simulink model "Model_OnlyDark_17_09_07_hperrorsign_manyouts"  (R2015a)
settings: Solver=FixedStepDiscrete  StartTime=0.0  StopTime=60  FixedStep=0.05  RelTol=1e-3
InitFcn:
  | %Ts=parameter.Ts;
  |    %Sampling Time, 50 times slower than original model
model workspace (MAT data in the model file):
  padsize = 8
  x1 = 14
undefined symbols (not defined in the file): alpha_downslope_off, alpha_downslope_on, alpha_upslope_off, alpha_upslope_on, fdsr_lp, hdegs, TimeStep, vdegs
libraries: visionfilter x3, visionutilities x3
settings Model: tstep=0.1  TimeStep=0.1  CovSFcnEnable=off  Creator=a1174239  LastModifiedBy=John
settings SolverCC: AlgebraicLoopSolver=LineSearch
settings DataIOCC: MaxDataPoints=1
settings OptimizationCC: ExpressionDepthLimit=2147483647  EfficientMapNaN2IntZero=off
settings DebuggingCC: UnderspecifiedInitializationDetection=Classic  MergeDetectMultiDrivingBlocksExec=none  SolverPrmCheckMsg=warning  MultiTaskDSMMsg=warning  MultiTaskCondExecSysMsg=none  ParameterPrecisionLossMsg=none  StateNameClashWarn=warning
settings HardwareCC: TargetLongLongMode=on  TargetIntDivRoundTo=Zero  TargetEndianess=LittleEndian  TargetHWDeviceType=MATLAB Host  ProdEqTarget=off
settings CodeAppCC: MaxIdLength=128
settings GRTTargetCC: CombineOutputUpdateFcns=off  GRTInterface=on

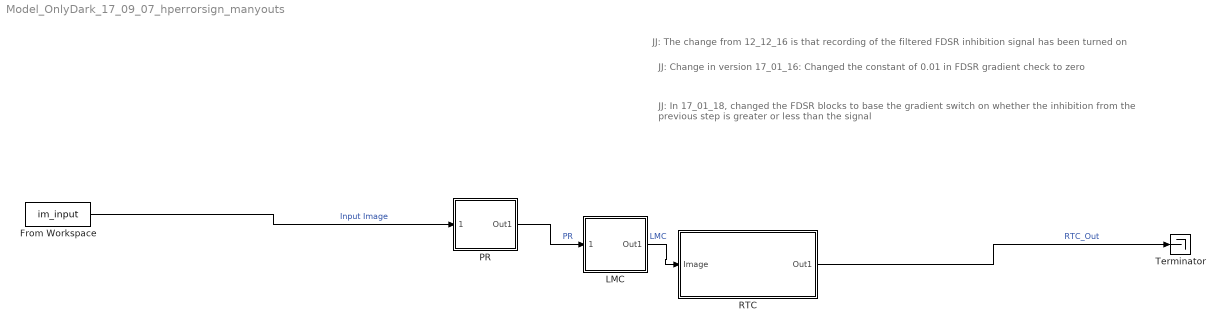
== system Model_OnlyDark_17_09_07_hperrorsign_manyouts ==
  note: JJ: In 17_01_18, changed the FDSR blocks to base the gradient switch on whether the inhibition from the previous step is greater or less than the signal
  note: JJ: Change in version 17_01_16: Changed the constant of 0.01 in FDSR gradient check to zero
  note: JJ: The change from 12_12_16 is that recording of the filtered FDSR inhibition signal has been turned on
  From Workspace : FromWorkspace  VariableName=im_input  SampleTime=0.001  Interpolate=off  OutputAfterFinalValue=Holding final value
  LMC : Subsystem
  PR : Subsystem
  RTC : Subsystem
  Terminator : Terminator
  wires:
  PR/1(Out1) -> LMC/1(Image)  "PR"
  LMC/1(Out1) -> RTC/1(Image)  "LMC"
  RTC/1(Out1) -> Terminator/1  "RTC_Out"
  From Workspace/1 -> PR/1(Image)  "Input Image"

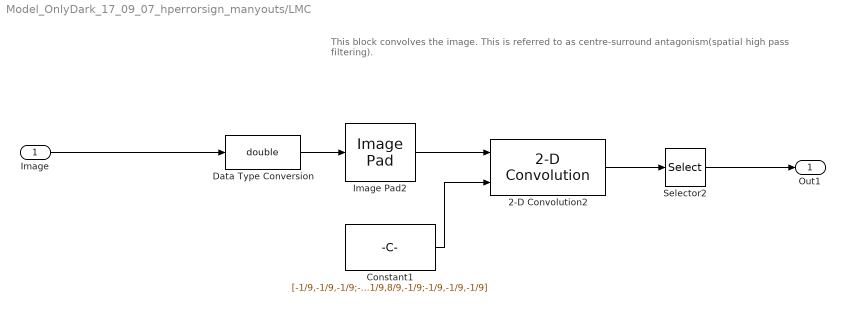
== system Model_OnlyDark_17_09_07_hperrorsign_manyouts/LMC ==
  note: This block convolves the image. This is referred to as centre-surround antagonism(spatial high pass filtering).
  Image : Inport
  2-D Convolution2 : visionfilter/2-D Convolution  outSize=Same as input port I1  normalize=off  outputMode=Binary point scaling  outputWordLength=32  outputFracLength=12  prodOutputMode=Binary point scaling  prodOutputWordLength=32  prodOutputFracLength=10  roundingMode=Floor  overflowMode=off
  Constant1 : Constant  Value=[-1/9,-1/9,-1/9;-1/9,8/9,-1/9;-1/9,-1/9,-1/9]
  Data Type Conversion : DataTypeConversion  OutDataTypeStr=double
  Image Pad2 : visionutilities/Image Pad  method=Symmetric  valSrc=Specify via dialog  value=0  spec=Pad size  rowDirection=Both left and right  outRowsMode=User-specified  rowSize=1  outColSize=10  colDirection=Both top and bottom  outColsMode=User-specified  colSize=1  outRowSize=12  trunc_flag=None
  Selector2 : Selector  NumberOfDimensions=2  InputPortWidth=3  IndexOptions=Index vector (dialog),Index vector (dialog)  Indices=[2:vdegs+1],[2:hdegs+1]  OutputSizes=1,1
  Out1 : Outport
  wires:
  Constant1/1 -> 2-D Convolution2/2
  Image Pad2/1 -> 2-D Convolution2/1
  2-D Convolution2/1 -> Selector2/1
  Selector2/1 -> Out1/1
  Image/1 -> Data Type Conversion/1
  Data Type Conversion/1 -> Image Pad2/1

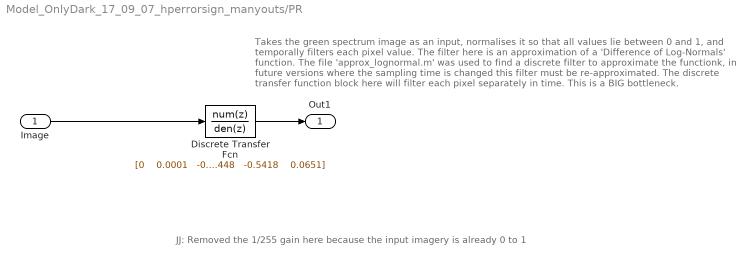
== system Model_OnlyDark_17_09_07_hperrorsign_manyouts/PR ==
  note: JJ: Removed the 1/255 gain here because the input imagery is already 0 to 1
  note: Takes the green spectrum image as an input, normalises it so that all values lie between 0
      | and 1, and temporally filters each pixel value. The filter here is an approximation of a
      | 'Difference of Log-Normals' function. The file 'approx_lognormal.m' was used to find a discrete
      | filter to approximate the functionk, in future versions where the sampling time is changed this filter
      | must be re-approximated.
      |
      | The discrete transfer function block here will filter each pixel separately in time. This is a BIG bottleneck.
  Image : Inport
  Discrete Transfer Fcn : DiscreteTransferFcn  Numerator="[0    0.0001   -0.0011    0.0052   -0.0170    0.0439   -0.0574    0.1789   -0.1524]"  Denominator="[ 1.0000   -4.3331    8.6847  -10.7116    9.0004   -5.3058    2.1448   -0.5418    0.0651]"
  Out1 : Outport
  wires:
  Image/1 -> Discrete Transfer Fcn/1
  Discrete Transfer Fcn/1 -> Out1/1

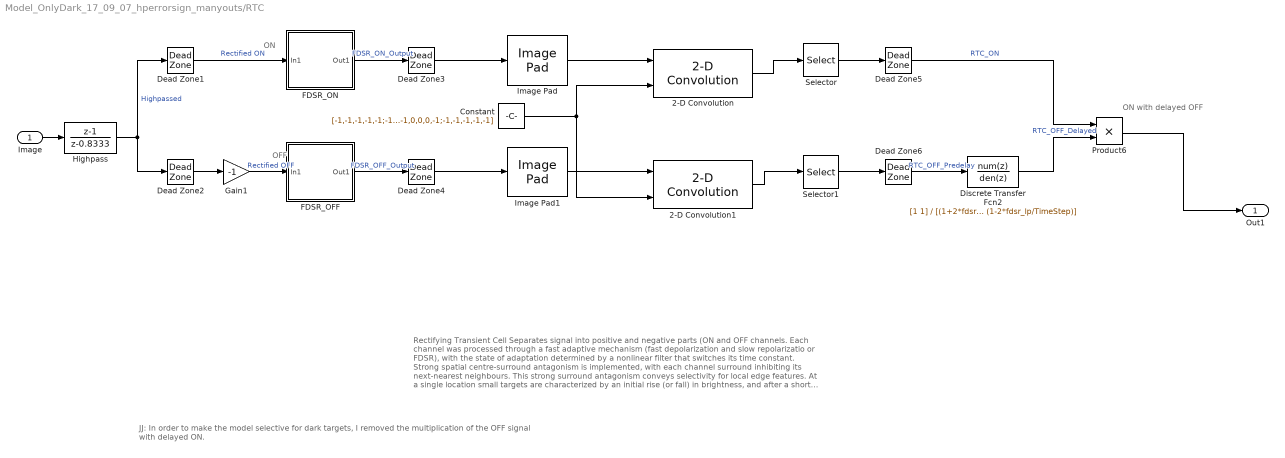
== system Model_OnlyDark_17_09_07_hperrorsign_manyouts/RTC ==
  note: ON with delayed OFF
  note: JJ: In order to make the model selective for dark targets, I removed the multiplication of the OFF signal with delayed ON.
  note: ON
  note: OFF
  note: Rectifying Transient Cell Separates signal into positive and negative parts (ON and OFF channels. Each channel was processed through a fast adaptive mechanism (fast depolarization and slow repolarizatio or FDSR),
      | with the state of adaptation determined by a nonlinear filter that switches its time constant. Strong spatial centre-surround antagonism is implemented, with each channel surround inhibiting its next-nearest neighbours.
      | This strong surround antagonism conveys selectivity for local edge features. At a single location small targets are characterized by an initial rise (or fall) in brightness, and after a short delay are followed by a corresponding
      | fall (or rise), irrespective of the direction of travel. Sensitivity to targets independent of their polarity was provided by multiplying each contrast channel (ON or OFF) with a delayed version of the opposite polarity
      | (via a low-pass filter,) and then summing the outputs.
  Image : Inport
  2-D Convolution : visionfilter/2-D Convolution  outSize=Same as input port I1  normalize=off  outputMode=Binary point scaling  outputWordLength=32  outputFracLength=12  prodOutputMode=Binary point scaling  prodOutputWordLength=32  prodOutputFracLength=10  roundingMode=Floor  overflowMode=off
  2-D Convolution1 : visionfilter/2-D Convolution  outSize=Same as input port I1  normalize=off  outputMode=Binary point scaling  outputWordLength=32  outputFracLength=12  prodOutputMode=Binary point scaling  prodOutputWordLength=32  prodOutputFracLength=10  roundingMode=Floor  overflowMode=off
  Constant : Constant  Value=[-1,-1,-1,-1,-1;-1,0,0,0,-1;-1,0,2,0,-1; -1,0,0,0,-1;-1,-1,-1,-1,-1]
  Dead Zone{1,3..6} (5 alike) : DeadZone  LowerValue=-inf  UpperValue=0  SaturateOnIntegerOverflow=on
  Dead Zone2 : DeadZone  LowerValue=0  UpperValue=inf  SaturateOnIntegerOverflow=on
  Discrete Transfer Fcn2 : DiscreteTransferFcn  Numerator=[1 1]  Denominator=[(1+2*fdsr_lp/TimeStep), (1-2*fdsr_lp/TimeStep)]
  FDSR_OFF : Subsystem
  FDSR_ON : Subsystem
  Gain1 : Gain  Gain=-1
  Highpass : DiscreteTransferFcn  Numerator=[1 -1]  Denominator=[1 -0.8333]
  Image Pad : visionutilities/Image Pad  method=Symmetric  valSrc=Specify via dialog  value=0  spec=Pad size  rowDirection=Both left and right  outRowsMode=User-specified  rowSize=2  outColSize=10  colDirection=Both top and bottom  outColsMode=User-specified  colSize=2  outRowSize=12  trunc_flag=None
  Image Pad1 : visionutilities/Image Pad  method=Symmetric  valSrc=Specify via dialog  value=0  spec=Pad size  rowDirection=Both left and right  outRowsMode=User-specified  rowSize=2  outColSize=10  colDirection=Both top and bottom  outColsMode=User-specified  colSize=2  outRowSize=12  trunc_flag=None
  Product6 : Product  RndMeth=Zero
  Selector : Selector  NumberOfDimensions=2  InputPortWidth=3  IndexOptions=Index vector (dialog),Index vector (dialog)  Indices=[3:vdegs+2],[3:hdegs+2]  OutputSizes=1,1
  Selector1 : Selector  NumberOfDimensions=2  InputPortWidth=3  IndexOptions=Index vector (dialog),Index vector (dialog)  Indices=[3:vdegs+2],[3:hdegs+2]  OutputSizes=1,1
  Out1 : Outport
  wires:
  Gain1/1 -> FDSR_OFF/1(In1)  "Rectified OFF"
  Discrete Transfer Fcn2/1 -> Product6/2  "RTC_OFF_Delayed"
  Dead Zone1/1 -> FDSR_ON/1(In1)  "Rectified ON"
  Dead Zone2/1 -> Gain1/1
  Dead Zone6/1 -> Discrete Transfer Fcn2/1  "RTC_OFF_Predelay"
  Dead Zone5/1 -> Product6/1  "RTC_ON"
  Image Pad/1 -> 2-D Convolution/1
  Constant/1 -> 2-D Convolution1/2, 2-D Convolution/2
  2-D Convolution/1 -> Selector/1
  Image Pad1/1 -> 2-D Convolution1/1
  2-D Convolution1/1 -> Selector1/1
  Dead Zone4/1 -> Image Pad1/1
  Dead Zone3/1 -> Image Pad/1
  Selector1/1 -> Dead Zone6/1
  Selector/1 -> Dead Zone5/1
  Product6/1 -> Out1/1
  FDSR_ON/1(Out1) -> Dead Zone3/1  "FDSR_ON_Output"
  FDSR_OFF/1(Out1) -> Dead Zone4/1  "FDSR_OFF_Output"
  Image/1 -> Highpass/1
  Highpass/1 -> Dead Zone2/1, Dead Zone1/1  "Highpassed"

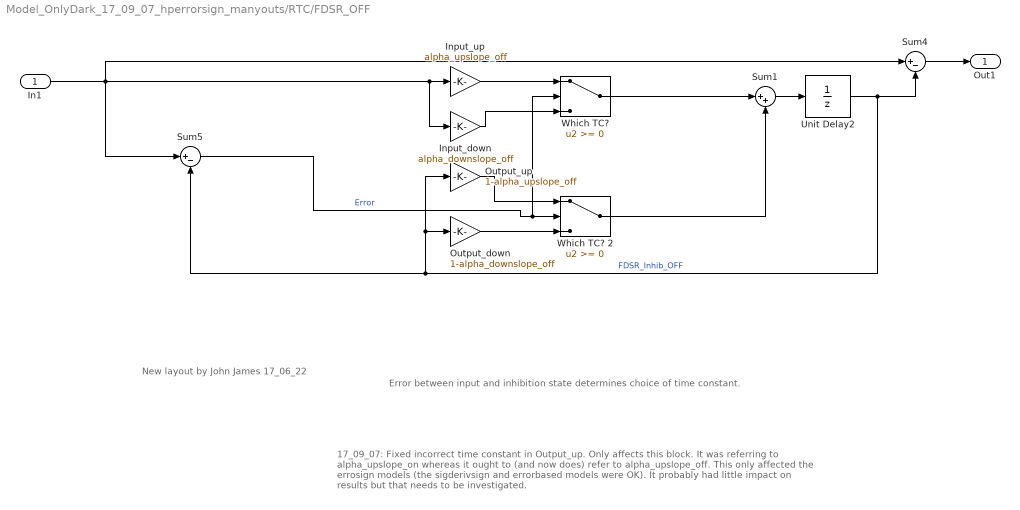
== system Model_OnlyDark_17_09_07_hperrorsign_manyouts/RTC/FDSR_OFF ==
  note: 17_09_07: Fixed incorrect time constant in Output_up. Only affects this block. It was referring to alpha_upslope_on whereas it ought to (and now does) refer to alpha_upslope_off.
      | This only affected the errosign models (the sigderivsign and errorbased models were OK). It probably had little impact on results but that needs to be investigated.
  note: Error between input and inhibition state determines choice of time constant.
  note: New layout by John James 17_06_22
  In1 : Inport
  Input_down : Gain  Gain=alpha_downslope_off
  Input_up : Gain  Gain=alpha_upslope_off
  Output_down : Gain  Gain=1-alpha_downslope_off
  Output_up : Gain  Gain=1-alpha_upslope_off
  Sum1 : Sum  Inputs=|++
  Sum4 : Sum  Inputs=|+-
  Sum5 : Sum  Inputs=|+-
  Unit Delay2 : UnitDelay  SampleTime=-1
  Which TC? : Switch
  Which TC? 2 : Switch
  Out1 : Outport
  wires:
  In1/1 -> Input_down/1, Input_up/1, Sum5/1, Sum4/1
  Input_up/1 -> Which TC?/1
  Input_down/1 -> Which TC?/3
  Output_up/1 -> Which TC? 2/1
  Output_down/1 -> Which TC? 2/3
  Which TC?/1 -> Sum1/1
  Which TC? 2/1 -> Sum1/2
  Sum4/1 -> Out1/1
  Sum1/1 -> Unit Delay2/1
  Unit Delay2/1 -> Sum5/2, Output_up/1, Output_down/1, Sum4/2  "FDSR_Inhib_OFF"
  Sum5/1 -> Which TC?/2, Which TC? 2/2  "Error"

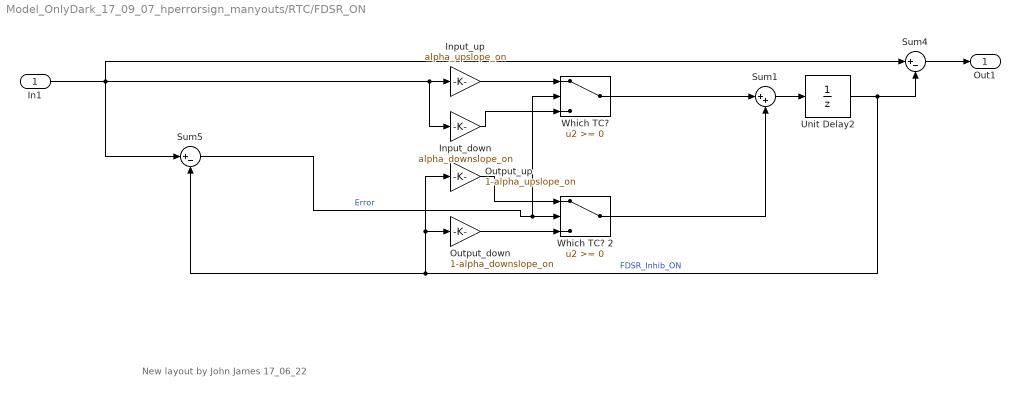
== system Model_OnlyDark_17_09_07_hperrorsign_manyouts/RTC/FDSR_ON ==
  note: New layout by John James 17_06_22
  In1 : Inport
  Input_down : Gain  Gain=alpha_downslope_on
  Input_up : Gain  Gain=alpha_upslope_on
  Output_down : Gain  Gain=1-alpha_downslope_on
  Output_up : Gain  Gain=1-alpha_upslope_on
  Sum1 : Sum  Inputs=|++
  Sum4 : Sum  Inputs=|+-
  Sum5 : Sum  Inputs=|+-
  Unit Delay2 : UnitDelay  SampleTime=-1
  Which TC? : Switch
  Which TC? 2 : Switch
  Out1 : Outport
  wires:
  In1/1 -> Input_down/1, Input_up/1, Sum5/1, Sum4/1
  Input_up/1 -> Which TC?/1
  Input_down/1 -> Which TC?/3
  Output_up/1 -> Which TC? 2/1
  Output_down/1 -> Which TC? 2/3
  Which TC?/1 -> Sum1/1
  Which TC? 2/1 -> Sum1/2
  Sum4/1 -> Out1/1
  Sum1/1 -> Unit Delay2/1
  Unit Delay2/1 -> Sum5/2, Output_up/1, Output_down/1, Sum4/2  "FDSR_Inhib_ON"
  Sum5/1 -> Which TC?/2, Which TC? 2/2  "Error"
